simulink model "SS"  (R2017a)
settings: Solver=VariableStepAuto  StartTime=0.0  StopTime=4100  RelTol=1e-3
values from neighbouring files (symbols this model uses):
  Ad = sysdd.A    [trock2.m]    (also in trock3.m)
  Bd2 = sysdd.B(1:2)/2    [trock3.m]
  Cd = sysdd.C    [trock2.m]    (also in trock3.m)
  Dd = -Dd    [trock2.m]    (also in trock3.m)
  Ed = sysdd.B(3:4)    [trock2.m]    (also in trock3.m)
  Kd = sysdd.D(:,3:4)    [trock2.m]    (also in trock3.m)
  Ts = 89.332338826894883    (= 89.3323388269)    [trock2.m]    (also in trock3.m = 8.93323388269)
libraries: simulink x1
settings Model: Creator=CBalla  LastModifiedBy=nvink

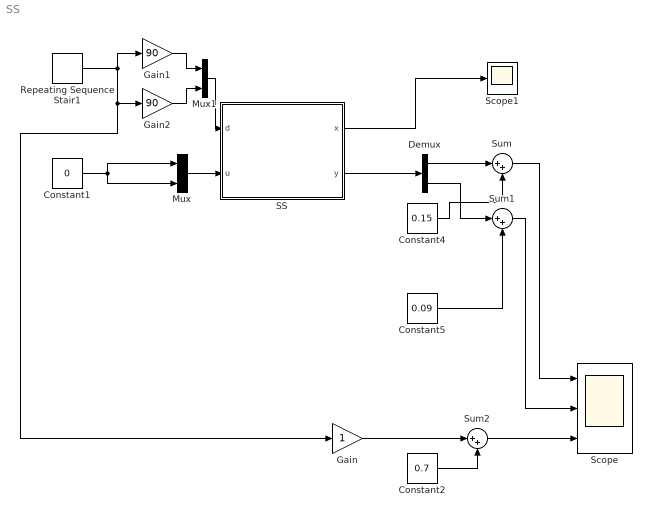
== system SS ==
  Constant1 : Constant  Value=0
  Constant2 : Constant  Value=0.7
  Constant4 : Constant  Value=0.15
  Constant5 : Constant  Value=0.09
  Demux : Demux  Outputs=2
  Gain : Gain
  Gain1 : Gain  Gain=90
  Gain2 : Gain  Gain=90
  Mux : Mux  Inputs=2
  Mux1 : Mux  Inputs=2
  Repeating Sequence Stair1 : simulink/Sources/Repeating Sequence Stair  OutValues=[-0.2 -0.1 0 0.1 0.2 0.3].'  tsamp=350  OutMin=[]  OutMax=[]  OutDataTypeStr=double  OutputDataTypeScalingMode=double  OutDataType=fixdt(0,8)  ConRadixGroup=Best Precision: Vector-wise  OutScaling=2^-12
  SS : Subsystem
  Scope : Scope  NumInputPorts=3
  Scope1 : Scope
  Sum : Sum  Inputs=|++
  Sum1 : Sum  Inputs=|++
  Sum2 : Sum  Inputs=|++
  wires:
  SS/1(x) -> Scope1/1
  Mux/1 -> SS/2(u)
  Mux1/1 -> SS/1(d)
  SS/2(y) -> Demux/1
  Demux/1 -> Sum/1
  Demux/2 -> Sum1/1
  Constant4/1 -> Sum/2
  Constant5/1 -> Sum1/2
  Sum/1 -> Scope/1
  Sum1/1 -> Scope/2
  Constant1/1 -> Mux/2, Mux/1
  Repeating Sequence Stair1/1 -> Gain2/1, Gain/1, Gain1/1
  Gain/1 -> Sum2/1
  Gain2/1 -> Mux1/2
  Gain1/1 -> Mux1/1
  Sum2/1 -> Scope/3
  Constant2/1 -> Sum2/2

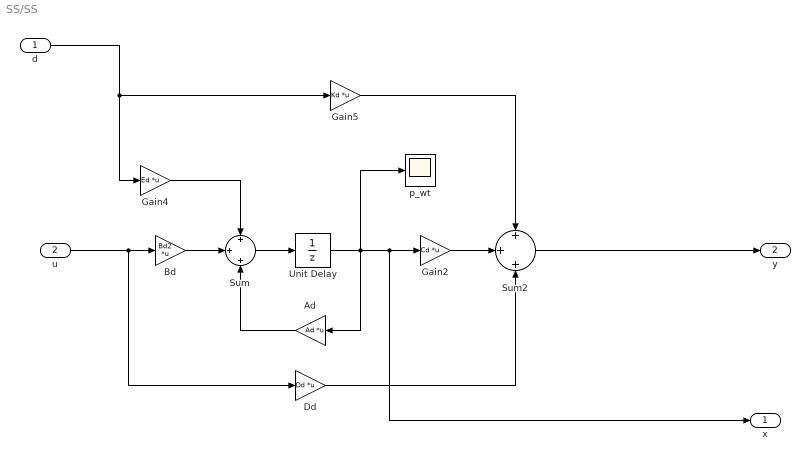
== system SS/SS ==
  d : Inport
  u : Inport  Port=2
  Ad : Gain  Gain=Ad  Multiplication=Matrix(K*u)
      mask Display:
      | %color('cyan')
      | color('magenta')
      | disp('{\bf\fontsize{14}Ad}', 'texmode','on');
      | %disp('Ad')
  Bd : Gain  Gain=Bd2  Multiplication=Matrix(K*u)
      mask Display:
      | %color('cyan')
      | color('magenta')
      | disp('{\bf\fontsize{14}Bd}', 'texmode','on');
      | %disp('Bd')
  Dd : Gain  Gain=Dd  Multiplication=Matrix(K*u)
      mask Display:
      | %color('cyan')
      | color('magenta')
      | disp('{\bf\fontsize{14}Dd}', 'texmode','on');
      | %disp('Dd')
  Gain2 : Gain  Gain=Cd  Multiplication=Matrix(K*u)
      mask Display:
      | %color('cyan')
      | color('magenta')
      | disp('{\bf\fontsize{14}Cd}', 'texmode','on');
      | %disp('Cd')
  Gain4 : Gain  Gain=Ed  Multiplication=Matrix(K*u)
      mask Display:
      | %color('cyan')
      | color('magenta')
      | disp('{\bf\fontsize{14}Ed}', 'texmode','on');
      | %disp('Ed')
  Gain5 : Gain  Gain=Kd  Multiplication=Matrix(K*u)
      mask Display:
      | %color('cyan')
      | color('magenta')
      | disp('{\bf\fontsize{14}Kd}', 'texmode','on');
      | %disp('Kd')
  Sum : Sum  Inputs=+|+|+
  Sum2 : Sum  Inputs=+|+|+
  Unit Delay : UnitDelay  SampleTime=Ts
  p_wt : Scope
  x : Outport
  y : Outport  Port=2
  wires:
  Sum2/1 -> y/1
  Sum/1 -> Unit Delay/1
  Bd/1 -> Sum/2
  Ad/1 -> Sum/3
  Unit Delay/1 -> p_wt/1, x/1, Gain2/1, Ad/1
  u/1 -> Dd/1, Bd/1
  d/1 -> Gain4/1, Gain5/1
  Gain2/1 -> Sum2/2
  Dd/1 -> Sum2/3
  Gain4/1 -> Sum/1
  Gain5/1 -> Sum2/1
